simulink model "hpt_v2_topology2_paper"  (R2025a)
settings: Solver=ode23tb  StartTime=0.0  StopTime=0.2  RelTol=1e-3
model workspace (MAT data in the model file):
  hpt_ctrl_Ts = 2e-05
  hpt_energy_bridge_polarity = -1
  hpt_energy_control_sign = -1
  hpt_energy_i_ki = 100
  hpt_energy_i_kp = 0.5
  hpt_energy_id_max = 20
  hpt_energy_vff_gain = 1.06
  hpt_grid_f0 = 50
  hpt_inj_phase_offset = -1.05
  hpt_m_energy = 0
  hpt_m_energy_max = 0.95
  hpt_m_reg = 0.1
  hpt_m_reg_max = 0.8
  hpt_pll_ki = 2500
  hpt_pll_kp = 80
  hpt_pwm_fs = 2000
  hpt_reg_openloop_amp = 0
  hpt_reg_openloop_phase = 0
  hpt_reg_polarity = 1
  hpt_s2_resistance = 0.001
  hpt_sac_actor_select_mode = 0
  hpt_sac_dynamic_reg_limit = 0.6
  hpt_sac_enable = 0
  hpt_sac_energy_enable = 0
  hpt_sac_energy_max = 0.95
  hpt_sac_fixed_energy_d = 0
  hpt_sac_fixed_energy_q = 0
  hpt_sac_fixed_reg_d = 0
  hpt_sac_fixed_reg_q = 0
  hpt_sac_guard_enable = 0
  hpt_sac_i_base_peak = 816.496580928
  hpt_sac_policy_mode = 0
  hpt_sac_reg_d_gain = 1
  hpt_sac_reg_max = 0.8
  hpt_sac_reg_polarity = 1
  hpt_sac_reg_q_gain = 1
  hpt_sac_topology_id = 2
  hpt_sac_vdc_ref = 800
  hpt_sac_vref_phase = 230
  hpt_swell_gain_scale = 1
  hpt_swell_m_reg_max = 0.5
  hpt_swell_phase_offset = -0.5
  hpt_vdc_ki = 0.2
  hpt_vdc_kp = 2
  hpt_vdc_ref = 800
  hpt_vref_lv = 207
  hpt_vreg_ki = 0
  hpt_vreg_kp = 20
libraries: spsSeriesRLCBranchLib x17, simulink x9, spsLinearTransformerLib x9, spsVoltageMeasurementLib x7, spsGroundLib x5, spsUniversalBridgeLib x4, spsThreePhaseVIMeasurementLib x3, spsIGBTLib x1, spsThreePhaseSourceLib x1, spsThreePhaseSeriesRLCLoadLib x1, spsThreePhaseSeriesRLCBranchLib x1, spspowerguiLib x1
(part 1 of 2)
settings Model: Creator=m1391  LastModifiedBy=m1391

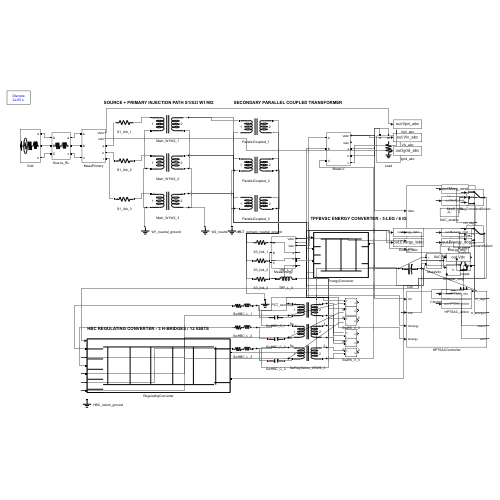
[thumbnail: Simulink's stored preview of the top-level diagram]
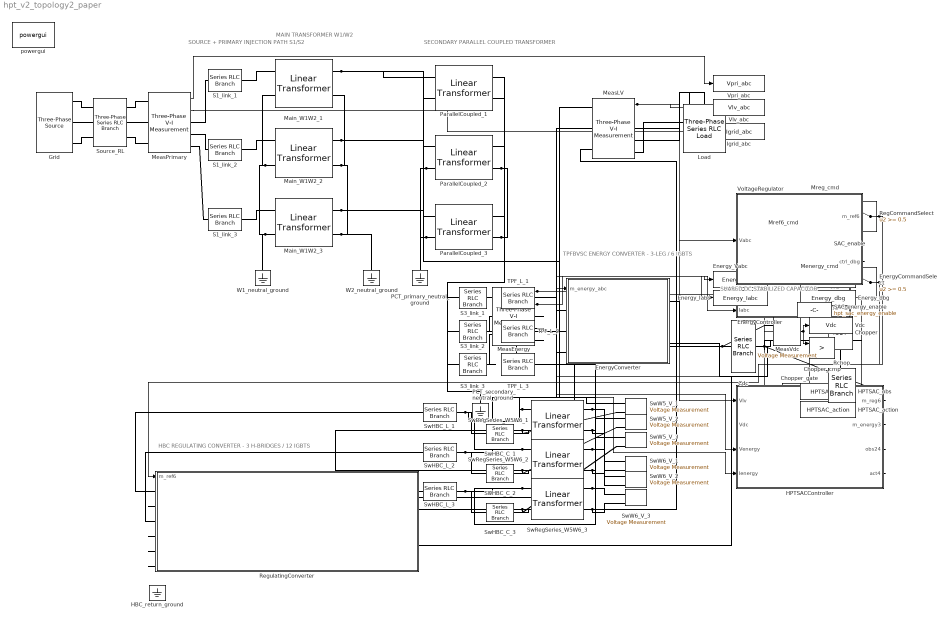
== system hpt_v2_topology2_paper ==
  note: SOURCE + PRIMARY INJECTION PATH S1/S2
  note: MAIN TRANSFORMER W1/W2
  note: SECONDARY PARALLEL COUPLED TRANSFORMER
  note: HBC REGULATING CONVERTER - 3 H-BRIDGES / 12 IGBTS
  note: TPFBVSC ENERGY CONVERTER - 3-LEG / 6 IGBTS
  note: SHARED DC STABILIZED CAPACITOR
  Cdc : spsSeriesRLCBranchLib/Series RLC Branch  LConnTagsString=__new0  RConnTagsString=__new0  BranchType=C  Resistance=1  Inductance=1e-3  SetiL0=off  InitialCurrent=0  Capacitance=0.0022  Setx0=on  InitialVoltage=800  Measurements=None
  Chopper : spsIGBTLib/IGBT  Ron=0.001  Lon=0  Vf=1  Tf=1e-6  Tt=2e-6  IC=0  Rs=1e5  Cs=inf  Measurements=on
  Chopper_cmp : RelationalOperator  Operator=>  OutDataTypeStr=boolean  RndMeth=Simplest  InputSameDT=off
  Chopper_gate : Constant  Value=850
  EnergyCommandSelect : Switch  Threshold=0.5  SaturateOnIntegerOverflow=off  InputSameDT=off
  EnergyController : Subsystem
  EnergyConverter : Subsystem
      mask Display:
      | color('black');
      | plot([10 90 90 10 10],[10 10 90 90 10]);
      | plot([20 80],[78 78]); plot([20 80],[22 22]);
      | plot([28 28],[22 78]); plot([50 50],[22 78]); plot([72 72],[22 78]);
      | plot([10 20],[65 65]); plot([10 20],[50 50]); plot([10 20],[35 35]);
      | plot([80 90],[65 65]); plot([80 90],[35 35]);
  Energy_Iabc : ToWorkspace  VariableName=Energy_Iabc  SampleTime=2e-05
  Energy_Vabc : ToWorkspace  VariableName=Energy_Vabc  SampleTime=2e-05
  Energy_dbg : ToWorkspace  VariableName=Energy_dbg  SampleTime=2e-05
  Grid : spsThreePhaseSourceLib/Three-Phase Source  InternalConnection=Yg  VoltagePhases=off  Voltage=10000  PhaseAngle=0  Voltage_phases=[25e3 25e3 25e3]/sqrt(3)  PhaseAngles_phases=[0 -120 +120]  Frequency=50  NonIdealSource=on  SpecifyImpedance=off  Resistance=0.8929  Inductance=16.58e-3  ShortCircuitLevel=100e6  BaseVoltage=25e3  XRratio=7  BusType=swing  Pref=10e3  Qref=0  Prefabc=[10e3, 10e3, 10e3]  Qrefabc=[0, 0, 0]  Qmin=-inf  Qmax=inf
  HBC_return_ground : spsGroundLib/Ground  LConnTagsString=a
  HPTSACController : Subsystem
  HPTSAC_action : ToWorkspace  VariableName=HPTSAC_action  SampleTime=2e-05
  HPTSAC_obs : ToWorkspace  VariableName=HPTSAC_obs  SampleTime=2e-05
  Igrid_abc : ToWorkspace  VariableName=Igrid_abc  SampleTime=2e-05
  Load : spsThreePhaseSeriesRLCLoadLib/Three-Phase Series RLC Load  LConnTagsString=A|B|C  Configuration=Y (grounded)  NominalVoltage=400  Vabc=[1e3 1e3 1e3]  Vabcp=[1e3 1e3 1e3]  NominalFrequency=50  UnbalancedPower=off  ActivePower=400000  InductivePower=0  CapacitivePower=0  Pabc=[10e3 9e3 11e3]  QLabc=[100 90 110]  QCabc=[100 90 110]  Pabcp=[10e3 9e3 11e3]  QLabcp=[100 90 110]  QCabcp=[100 90 110]  Measurements=None  LoadType=constant Z
  Main_W1W2_1 : spsLinearTransformerLib/Linear Transformer  UNITS=pu  NominalPower=[133333.3333,50]  winding1=[5773.5027,0.005,0.025]  winding2=[230.9401,0.005,0.025]  ThreeWindings=off  winding3=[ 315e3 0.002 0.08 ]  RmLm=[ 500 500 ]  Measurements=None  DataType=off
  Main_W1W2_2 : spsLinearTransformerLib/Linear Transformer  UNITS=pu  NominalPower=[133333.3333,50]  winding1=[5773.5027,0.005,0.025]  winding2=[230.9401,0.005,0.025]  ThreeWindings=off  winding3=[ 315e3 0.002 0.08 ]  RmLm=[ 500 500 ]  Measurements=None  DataType=off
  Main_W1W2_3 : spsLinearTransformerLib/Linear Transformer  UNITS=pu  NominalPower=[133333.3333,50]  winding1=[5773.5027,0.005,0.025]  winding2=[230.9401,0.005,0.025]  ThreeWindings=off  winding3=[ 315e3 0.002 0.08 ]  RmLm=[ 500 500 ]  Measurements=None  DataType=off
  MeasEnergy : spsThreePhaseVIMeasurementLib/Three-Phase V-I Measurement  VoltageMeasurement=phase-to-ground  SetLabelV=off  LabelV=Vabc  Vpu=off  VpuLL=off  CurrentMeasurement=yes  SetLabelI=off  LabelI=Iabc  Ipu=off  Pbase=100e6  Vbase=500e3  OutputType=Complex  PhasorSimulation=off  PSBequivalent=0
  MeasLV : spsThreePhaseVIMeasurementLib/Three-Phase V-I Measurement  VoltageMeasurement=phase-to-ground  SetLabelV=off  LabelV=Vabc  Vpu=off  VpuLL=off  CurrentMeasurement=yes  SetLabelI=off  LabelI=Iabc  Ipu=off  Pbase=100e6  Vbase=500e3  OutputType=Complex  PhasorSimulation=off  PSBequivalent=0
  MeasPrimary : spsThreePhaseVIMeasurementLib/Three-Phase V-I Measurement  VoltageMeasurement=phase-to-ground  SetLabelV=off  LabelV=Vabc  Vpu=off  VpuLL=off  CurrentMeasurement=yes  SetLabelI=off  LabelI=Iabc  Ipu=off  Pbase=100e6  Vbase=500e3  OutputType=Complex  PhasorSimulation=off  PSBequivalent=0
  MeasVdc : spsVoltageMeasurementLib/Voltage Measurement  PhasorSimulation=off  OutputType=Complex  PSBequivalent=0
  Menergy_cmd : ToWorkspace  VariableName=Menergy_cmd  SampleTime=2e-05
  Mref6_cmd : ToWorkspace  VariableName=Mref6_cmd  SampleTime=2e-05
  Mreg_cmd : ToWorkspace  VariableName=Mreg_cmd  SampleTime=2e-05
  PCT_primary_neutral_ground : spsGroundLib/Ground  LConnTagsString=a
  PCT_secondary_neutral_ground : spsGroundLib/Ground  LConnTagsString=a
  ParallelCoupled_1 : spsLinearTransformerLib/Linear Transformer  UNITS=pu  NominalPower=[40000,50]  winding1=[230.9401,0.004,0.02]  winding2=[230.9401,0.004,0.02]  ThreeWindings=off  winding3=[ 315e3 0.002 0.08 ]  RmLm=[ 500 500 ]  Measurements=None  DataType=off
  ParallelCoupled_2 : spsLinearTransformerLib/Linear Transformer  UNITS=pu  NominalPower=[40000,50]  winding1=[230.9401,0.004,0.02]  winding2=[230.9401,0.004,0.02]  ThreeWindings=off  winding3=[ 315e3 0.002 0.08 ]  RmLm=[ 500 500 ]  Measurements=None  DataType=off
  ParallelCoupled_3 : spsLinearTransformerLib/Linear Transformer  UNITS=pu  NominalPower=[40000,50]  winding1=[230.9401,0.004,0.02]  winding2=[230.9401,0.004,0.02]  ThreeWindings=off  winding3=[ 315e3 0.002 0.08 ]  RmLm=[ 500 500 ]  Measurements=None  DataType=off
  Rchop : spsSeriesRLCBranchLib/Series RLC Branch  LConnTagsString=__new0  RConnTagsString=__new0  BranchType=R  Resistance=5.3333  Inductance=1e-3  SetiL0=off  InitialCurrent=0  Capacitance=1e-6  Setx0=off  InitialVoltage=0  Measurements=None
  RegCommandSelect : Switch  Threshold=0.5  SaturateOnIntegerOverflow=off  InputSameDT=off
  RegulatingConverter : Subsystem
      mask Display:
      | color('black');
      | plot([5 95 95 5 5],[10 10 90 90 10]);
      | plot([15 85],[78 78]); plot([15 85],[22 22]);
      | plot([18 18],[22 78]); plot([32 32],[22 78]);
      | plot([45 45],[22 78]); plot([59 59],[22 78]);
      | plot([72 72],[22 78]); plot([86 86],[22 78]);
      | plot([5 15],[75 75]); plot([5 15],[60 60]); plot([5 15],[45 45]);
      | plot([5 15],[30 30]); plot([5 15],[15 15]); plot([5 15],[10 10]);
      | plot([85 95],[75 75]); plot([85 95],[25 25]);
  S1_link_1 : spsSeriesRLCBranchLib/Series RLC Branch  LConnTagsString=__new0  RConnTagsString=__new0  BranchType=R  Resistance=1e-3  Inductance=1e-3  SetiL0=off  InitialCurrent=0  Capacitance=1e-6  Setx0=off  InitialVoltage=0  Measurements=None
  S1_link_2 : spsSeriesRLCBranchLib/Series RLC Branch  LConnTagsString=__new0  RConnTagsString=__new0  BranchType=R  Resistance=1e-3  Inductance=1e-3  SetiL0=off  InitialCurrent=0  Capacitance=1e-6  Setx0=off  InitialVoltage=0  Measurements=None
  S1_link_3 : spsSeriesRLCBranchLib/Series RLC Branch  LConnTagsString=__new0  RConnTagsString=__new0  BranchType=R  Resistance=1e-3  Inductance=1e-3  SetiL0=off  InitialCurrent=0  Capacitance=1e-6  Setx0=off  InitialVoltage=0  Measurements=None
  S3_link_1 : spsSeriesRLCBranchLib/Series RLC Branch  LConnTagsString=__new0  RConnTagsString=__new0  BranchType=R  Resistance=1e-3  Inductance=1e-3  SetiL0=off  InitialCurrent=0  Capacitance=1e-6  Setx0=off  InitialVoltage=0  Measurements=None
  S3_link_2 : spsSeriesRLCBranchLib/Series RLC Branch  LConnTagsString=__new0  RConnTagsString=__new0  BranchType=R  Resistance=1e-3  Inductance=1e-3  SetiL0=off  InitialCurrent=0  Capacitance=1e-6  Setx0=off  InitialVoltage=0  Measurements=None
  S3_link_3 : spsSeriesRLCBranchLib/Series RLC Branch  LConnTagsString=__new0  RConnTagsString=__new0  BranchType=R  Resistance=1e-3  Inductance=1e-3  SetiL0=off  InitialCurrent=0  Capacitance=1e-6  Setx0=off  InitialVoltage=0  Measurements=None
  SAC_enable : Constant  Value=hpt_sac_enable
  SAC_energy_enable : Constant  Value=hpt_sac_energy_enable
  Source_RL : spsThreePhaseSeriesRLCBranchLib/Three-Phase Series RLC Branch  LConnTagsString=A|B|C  RConnTagsString=A|B|C  BranchType=RL  Resistance=11.7851  Inductance=0.26259  Capacitance=1e-6  Measurements=None
  SwHBC_C_1 : spsSeriesRLCBranchLib/Series RLC Branch  LConnTagsString=__new0  RConnTagsString=__new0  BranchType=C  Resistance=1  Inductance=1e-3  SetiL0=off  InitialCurrent=0  Capacitance=2e-05  Setx0=off  InitialVoltage=0  Measurements=None
  SwHBC_C_2 : spsSeriesRLCBranchLib/Series RLC Branch  LConnTagsString=__new0  RConnTagsString=__new0  BranchType=C  Resistance=1  Inductance=1e-3  SetiL0=off  InitialCurrent=0  Capacitance=2e-05  Setx0=off  InitialVoltage=0  Measurements=None
  SwHBC_C_3 : spsSeriesRLCBranchLib/Series RLC Branch  LConnTagsString=__new0  RConnTagsString=__new0  BranchType=C  Resistance=1  Inductance=1e-3  SetiL0=off  InitialCurrent=0  Capacitance=2e-05  Setx0=off  InitialVoltage=0  Measurements=None
  SwHBC_L_1 : spsSeriesRLCBranchLib/Series RLC Branch  LConnTagsString=__new0  RConnTagsString=__new0  BranchType=RL  Resistance=0.03  Inductance=0.002  SetiL0=off  InitialCurrent=0  Capacitance=1e-6  Setx0=off  InitialVoltage=0  Measurements=None
  SwHBC_L_2 : spsSeriesRLCBranchLib/Series RLC Branch  LConnTagsString=__new0  RConnTagsString=__new0  BranchType=RL  Resistance=0.03  Inductance=0.002  SetiL0=off  InitialCurrent=0  Capacitance=1e-6  Setx0=off  InitialVoltage=0  Measurements=None
  SwHBC_L_3 : spsSeriesRLCBranchLib/Series RLC Branch  LConnTagsString=__new0  RConnTagsString=__new0  BranchType=RL  Resistance=0.03  Inductance=0.002  SetiL0=off  InitialCurrent=0  Capacitance=1e-6  Setx0=off  InitialVoltage=0  Measurements=None
  SwRegSeries_W5W6_1 : spsLinearTransformerLib/Linear Transformer  UNITS=pu  NominalPower=[30000,50]  winding1=[400,0.002,0.03]  winding2=[100,0.002,0.03]  ThreeWindings=off  winding3=[ 315e3 0.002 0.08 ]  RmLm=[ 500 500 ]  Measurements=None  DataType=off
  SwRegSeries_W5W6_2 : spsLinearTransformerLib/Linear Transformer  UNITS=pu  NominalPower=[30000,50]  winding1=[400,0.002,0.03]  winding2=[100,0.002,0.03]  ThreeWindings=off  winding3=[ 315e3 0.002 0.08 ]  RmLm=[ 500 500 ]  Measurements=None  DataType=off
  SwRegSeries_W5W6_3 : spsLinearTransformerLib/Linear Transformer  UNITS=pu  NominalPower=[30000,50]  winding1=[400,0.002,0.03]  winding2=[100,0.002,0.03]  ThreeWindings=off  winding3=[ 315e3 0.002 0.08 ]  RmLm=[ 500 500 ]  Measurements=None  DataType=off
  SwW5_V_1 : spsVoltageMeasurementLib/Voltage Measurement  PhasorSimulation=off  OutputType=Complex  PSBequivalent=0
  SwW5_V_2 : spsVoltageMeasurementLib/Voltage Measurement  PhasorSimulation=off  OutputType=Complex  PSBequivalent=0
  SwW5_V_3 : spsVoltageMeasurementLib/Voltage Measurement  PhasorSimulation=off  OutputType=Complex  PSBequivalent=0
  SwW6_V_1 : spsVoltageMeasurementLib/Voltage Measurement  PhasorSimulation=off  OutputType=Complex  PSBequivalent=0
  SwW6_V_2 : spsVoltageMeasurementLib/Voltage Measurement  PhasorSimulation=off  OutputType=Complex  PSBequivalent=0
  SwW6_V_3 : spsVoltageMeasurementLib/Voltage Measurement  PhasorSimulation=off  OutputType=Complex  PSBequivalent=0
  TPF_L_1 : spsSeriesRLCBranchLib/Series RLC Branch  LConnTagsString=__new0  RConnTagsString=__new0  BranchType=L  Resistance=1  Inductance=0.0015  SetiL0=off  InitialCurrent=0  Capacitance=1e-6  Setx0=off  InitialVoltage=0  Measurements=None
  TPF_L_2 : spsSeriesRLCBranchLib/Series RLC Branch  LConnTagsString=__new0  RConnTagsString=__new0  BranchType=L  Resistance=1  Inductance=0.0015  SetiL0=off  InitialCurrent=0  Capacitance=1e-6  Setx0=off  InitialVoltage=0  Measurements=None
  TPF_L_3 : spsSeriesRLCBranchLib/Series RLC Branch  LConnTagsString=__new0  RConnTagsString=__new0  BranchType=L  Resistance=1  Inductance=0.0015  SetiL0=off  InitialCurrent=0  Capacitance=1e-6  Setx0=off  InitialVoltage=0  Measurements=None
  Vdc : ToWorkspace  VariableName=Vdc  SampleTime=2e-05
  Vlv_abc : ToWorkspace  VariableName=Vlv_abc  SampleTime=2e-05
  VoltageRegulator : Subsystem
  Vpri_abc : ToWorkspace  VariableName=Vpri_abc  SampleTime=2e-05
  W1_neutral_ground : spsGroundLib/Ground  LConnTagsString=a
  W2_neutral_ground : spsGroundLib/Ground  LConnTagsString=a
  powergui : spspowerguiLib/powergui  Priority=1  SimulationMode=Discrete  SampleTime=2e-05  frequency=60  Iterations=50  frequencyindice=60  Pbase=100e6  ErrMax=1e-4  UnitsV=kV  UnitsW=MW  buscounter=0  FunctionMessages=off  echomessages=off  EnableUseOfTLC=off  CurrentSourceSwitches=off  DisableSnubberDevices=off  DisableRonSwitches=off  DisableVfSwitches=off  DisplayEquations=off  AutomaticDiscreteSolvers=off  SolverType=Tustin/Backward Euler (TBE)  Interpol=off  ExternalGateDelay=off  methode=off  Ts=100  x0status=blocks  SPID=on  SwTol=0  HookPort=off  NonlinearTolerance=1e-4  nMaxIteration=100  ContinueOnMaxIteration=off  RestoreLinks=warning  ResistiveCurrentMeasurement=off  Frange=[0:2:500]  Ylog=off  Xlog=on  ShowGrid=off  save=off  variable=ZData  structure=0  ZoomFFT=off  StartTime=0.0  cycles=1  DisplayStyle=1  fundamental=60  FreqAxis=off  MaxFrequency=1000  frequencyindicesteady=1  RmsSteady=1  display=off
  wires:
  MeasVdc/1 -> Chopper_cmp/1, Vdc/1, HPTSACController/2(Vdc), EnergyController/1(Vdc)
  Chopper_gate/1 -> Chopper_cmp/2
  Chopper_cmp/1 -> Chopper/1
  MeasPrimary/1 -> Vpri_abc/1
  MeasPrimary/2 -> Igrid_abc/1
  MeasLV/1 -> Vlv_abc/1, VoltageRegulator/1(Vabc), HPTSACController/1(Vlv)
  VoltageRegulator/1(m_ref6) -> RegCommandSelect/3
  HPTSACController/1(m_reg6) -> RegCommandSelect/1
  SAC_enable/1 -> RegCommandSelect/2
  RegCommandSelect/1 -> RegulatingConverter/1(m_ref6), Mref6_cmd/1
  VoltageRegulator/2(ctrl_dbg) -> Mreg_cmd/1
  MeasEnergy/1 -> EnergyController/2(Vabc), HPTSACController/3(Venergy), Energy_Vabc/1
  MeasEnergy/2 -> EnergyController/3(Iabc), HPTSACController/4(Ienergy), Energy_Iabc/1
  EnergyController/1(m_energy_abc) -> EnergyCommandSelect/3
  HPTSACController/2(m_energy3) -> EnergyCommandSelect/1
  SAC_energy_enable/1 -> EnergyCommandSelect/2
  EnergyCommandSelect/1 -> EnergyConverter/1(m_energy_abc), Menergy_cmd/1
  EnergyController/2(energy_dbg) -> Energy_dbg/1
  HPTSACController/3(obs24) -> HPTSAC_obs/1
  HPTSACController/4(act4) -> HPTSAC_action/1
  connections:
  Grid/RConn1 -- Source_RL/LConn1
  Source_RL/RConn1 -- MeasPrimary/LConn1
  MeasPrimary/RConn1 -- S1_link_1/LConn1
  S1_link_1/RConn1 -- Main_W1W2_1/LConn1
  ParallelCoupled_1/LConn1 -- Main_W1W2_1/RConn1 -- SwRegSeries_W5W6_1/RConn1 -- SwW6_V_1/LConn1
  MeasLV/LConn1 -- SwRegSeries_W5W6_1/RConn2 -- SwW6_V_1/LConn2
  MeasLV/RConn1 -- Load/LConn1
  ParallelCoupled_1/RConn1 -- S3_link_1/LConn1
  S3_link_1/RConn1 -- MeasEnergy/LConn1
  MeasEnergy/RConn1 -- TPF_L_1/LConn1
  TPF_L_1/RConn1 -- EnergyConverter/LConn1
  RegulatingConverter/LConn1 -- SwHBC_L_1/LConn1
  SwHBC_L_1/RConn1 -- SwHBC_C_1/LConn1 -- SwRegSeries_W5W6_1/LConn1 -- SwW5_V_1/LConn1
  RegulatingConverter/LConn2 -- SwHBC_C_1/RConn1 -- SwRegSeries_W5W6_1/LConn2 -- SwW5_V_1/LConn2
  Grid/RConn2 -- Source_RL/LConn2
  Source_RL/RConn2 -- MeasPrimary/LConn2
  MeasPrimary/RConn2 -- S1_link_2/LConn1
  S1_link_2/RConn1 -- Main_W1W2_2/LConn1
  ParallelCoupled_2/LConn1 -- Main_W1W2_2/RConn1 -- SwRegSeries_W5W6_2/RConn1 -- SwW6_V_2/LConn1
  MeasLV/LConn2 -- SwRegSeries_W5W6_2/RConn2 -- SwW6_V_2/LConn2
  MeasLV/RConn2 -- Load/LConn2
  ParallelCoupled_2/RConn1 -- S3_link_2/LConn1
  S3_link_2/RConn1 -- MeasEnergy/LConn2
  MeasEnergy/RConn2 -- TPF_L_2/LConn1
  TPF_L_2/RConn1 -- EnergyConverter/LConn2
  RegulatingConverter/LConn3 -- SwHBC_L_2/LConn1
  SwHBC_L_2/RConn1 -- SwHBC_C_2/LConn1 -- SwRegSeries_W5W6_2/LConn1 -- SwW5_V_2/LConn1
  RegulatingConverter/LConn4 -- SwHBC_C_2/RConn1 -- SwRegSeries_W5W6_2/LConn2 -- SwW5_V_2/LConn2
  Grid/RConn3 -- Source_RL/LConn3
  Source_RL/RConn3 -- MeasPrimary/LConn3
  MeasPrimary/RConn3 -- S1_link_3/LConn1
  S1_link_3/RConn1 -- Main_W1W2_3/LConn1
  ParallelCoupled_3/LConn1 -- Main_W1W2_3/RConn1 -- SwRegSeries_W5W6_3/RConn1 -- SwW6_V_3/LConn1
  MeasLV/LConn3 -- SwRegSeries_W5W6_3/RConn2 -- SwW6_V_3/LConn2
  MeasLV/RConn3 -- Load/LConn3
  ParallelCoupled_3/RConn1 -- S3_link_3/LConn1
  S3_link_3/RConn1 -- MeasEnergy/LConn3
  MeasEnergy/RConn3 -- TPF_L_3/LConn1
  TPF_L_3/RConn1 -- EnergyConverter/LConn3
  RegulatingConverter/LConn5 -- SwHBC_L_3/LConn1
  SwHBC_L_3/RConn1 -- SwHBC_C_3/LConn1 -- SwRegSeries_W5W6_3/LConn1 -- SwW5_V_3/LConn1
  RegulatingConverter/LConn6 -- SwHBC_C_3/RConn1 -- SwRegSeries_W5W6_3/LConn2 -- SwW5_V_3/LConn2
  Main_W1W2_2/LConn2 -- Main_W1W2_1/LConn2 -- Main_W1W2_3/LConn2 -- W1_neutral_ground/LConn1
  Main_W1W2_2/RConn2 -- Main_W1W2_1/RConn2 -- Main_W1W2_3/RConn2 -- W2_neutral_ground/LConn1
  ParallelCoupled_2/LConn2 -- ParallelCoupled_1/LConn2 -- ParallelCoupled_3/LConn2 -- PCT_primary_neutral_ground/LConn1
  ParallelCoupled_2/RConn2 -- ParallelCoupled_1/RConn2 -- ParallelCoupled_3/RConn2 -- PCT_secondary_neutral_ground/LConn1
  EnergyConverter/RConn1 -- Cdc/LConn1 -- RegulatingConverter/RConn1 -- MeasVdc/LConn1 -- Chopper/LConn1
  EnergyConverter/RConn2 -- RegulatingConverter/RConn2 -- MeasVdc/LConn2 -- Cdc/RConn1 -- Rchop/RConn1
  Chopper/RConn1 -- Rchop/LConn1

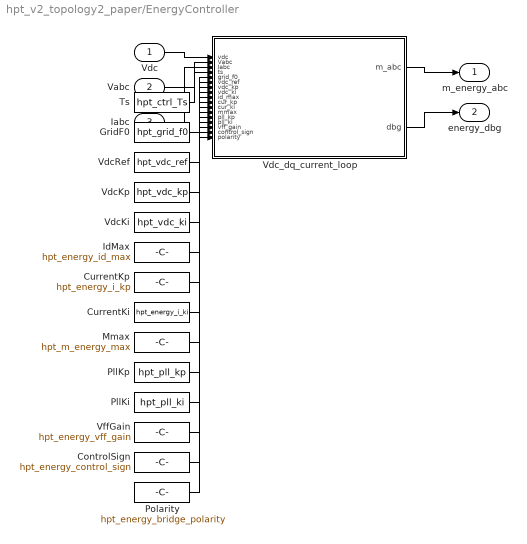
== system hpt_v2_topology2_paper/EnergyController ==
  Vdc : Inport
  Vabc : Inport  Port=2
  Iabc : Inport  Port=3
  ControlSign : Constant  Value=hpt_energy_control_sign
  CurrentKi : Constant  Value=hpt_energy_i_ki
  CurrentKp : Constant  Value=hpt_energy_i_kp
  GridF0 : Constant  Value=hpt_grid_f0
  IdMax : Constant  Value=hpt_energy_id_max
  Mmax : Constant  Value=hpt_m_energy_max
  PllKi : Constant  Value=hpt_pll_ki
  PllKp : Constant  Value=hpt_pll_kp
  Polarity : Constant  Value=hpt_energy_bridge_polarity
  Ts : Constant  Value=hpt_ctrl_Ts
  VdcKi : Constant  Value=hpt_vdc_ki
  VdcKp : Constant  Value=hpt_vdc_kp
  VdcRef : Constant  Value=hpt_vdc_ref
  Vdc_dq_current_loop : MATLAB Function  TreatAsAtomicUnit=on
  VffGain : Constant  Value=hpt_energy_vff_gain
  m_energy_abc : Outport
  energy_dbg : Outport  Port=2
  wires:
  Ts/1 -> Vdc_dq_current_loop/4(ts)
  GridF0/1 -> Vdc_dq_current_loop/5(grid_f0)
  VdcRef/1 -> Vdc_dq_current_loop/6(vdc_ref)
  VdcKp/1 -> Vdc_dq_current_loop/7(vdc_kp)
  VdcKi/1 -> Vdc_dq_current_loop/8(vdc_ki)
  IdMax/1 -> Vdc_dq_current_loop/9(id_max)
  CurrentKp/1 -> Vdc_dq_current_loop/10(cur_kp)
  CurrentKi/1 -> Vdc_dq_current_loop/11(cur_ki)
  Mmax/1 -> Vdc_dq_current_loop/12(mmax)
  PllKp/1 -> Vdc_dq_current_loop/13(pll_kp)
  PllKi/1 -> Vdc_dq_current_loop/14(pll_ki)
  VffGain/1 -> Vdc_dq_current_loop/15(vff_gain)
  ControlSign/1 -> Vdc_dq_current_loop/16(control_sign)
  Polarity/1 -> Vdc_dq_current_loop/17(polarity)
  Vdc/1 -> Vdc_dq_current_loop/1(vdc)
  Vabc/1 -> Vdc_dq_current_loop/2(Vabc)
  Iabc/1 -> Vdc_dq_current_loop/3(Iabc)
  Vdc_dq_current_loop/1(m_abc) -> m_energy_abc/1
  Vdc_dq_current_loop/2(dbg) -> energy_dbg/1

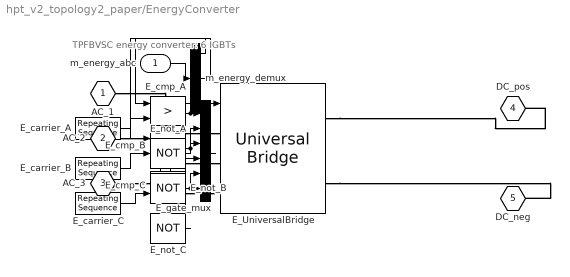
== system hpt_v2_topology2_paper/EnergyConverter ==
  note: TPFBVSC energy converter: 6 IGBTs
  m_energy_abc : Inport
  E_UniversalBridge : spsUniversalBridgeLib/Universal Bridge  Arms=3  SnubberResistance=1e5  SnubberCapacitance=inf  Device=IGBT / Diodes  Ron=1e-3  Lon=0  ForwardVoltages=[0.8 0.8]  ForwardVoltage=0  GTOparameters=[ 10e-6 , 20e-6 ]  IGBTparameters=[ 1e-6 , 2e-6 ]  Measurements=None  Measurements_2=None  converterType=Rectifier
  E_carrier_A : simulink/Sources/Repeating Sequence  rep_seq_t=[0 0.5/hpt_pwm_fs 1/hpt_pwm_fs]  rep_seq_y=[-1 1 -1]
  E_carrier_B : simulink/Sources/Repeating Sequence  rep_seq_t=[0 0.5/hpt_pwm_fs 1/hpt_pwm_fs]  rep_seq_y=[-1 1 -1]
  E_carrier_C : simulink/Sources/Repeating Sequence  rep_seq_t=[0 0.5/hpt_pwm_fs 1/hpt_pwm_fs]  rep_seq_y=[-1 1 -1]
  E_cmp_A : RelationalOperator  Operator=>  OutDataTypeStr=boolean  RndMeth=Simplest  InputSameDT=off
  E_cmp_B : RelationalOperator  Operator=>  OutDataTypeStr=boolean  RndMeth=Simplest  InputSameDT=off
  E_cmp_C : RelationalOperator  Operator=>  OutDataTypeStr=boolean  RndMeth=Simplest  InputSameDT=off
  E_gate_mux : Mux  Inputs=6
  E_not_A : Logic  Operator=NOT  AllPortsSameDT=off  OutDataTypeStr=boolean
  E_not_B : Logic  Operator=NOT  AllPortsSameDT=off  OutDataTypeStr=boolean
  E_not_C : Logic  Operator=NOT  AllPortsSameDT=off  OutDataTypeStr=boolean
  m_energy_demux : Demux  Outputs=3
  AC_1 : PMIOPort  Side=Left
  AC_2 : PMIOPort  Port=2  Side=Left
  AC_3 : PMIOPort  Port=3  Side=Left
  DC_pos : PMIOPort  Port=4  Side=Right
  DC_neg : PMIOPort  Port=5  Side=Right
  wires:
  m_energy_abc/1 -> m_energy_demux/1
  m_energy_demux/1 -> E_cmp_A/1
  E_carrier_A/1 -> E_cmp_A/2
  E_cmp_A/1 -> E_gate_mux/1, E_not_A/1
  E_not_A/1 -> E_gate_mux/2
  m_energy_demux/2 -> E_cmp_B/1
  E_carrier_B/1 -> E_cmp_B/2
  E_cmp_B/1 -> E_gate_mux/3, E_not_B/1
  E_not_B/1 -> E_gate_mux/4
  m_energy_demux/3 -> E_cmp_C/1
  E_carrier_C/1 -> E_cmp_C/2
  E_cmp_C/1 -> E_gate_mux/5, E_not_C/1
  E_not_C/1 -> E_gate_mux/6
  E_gate_mux/1 -> E_UniversalBridge/1
  connections:
  AC_1/RConn1 -- E_UniversalBridge/LConn1
  AC_2/RConn1 -- E_UniversalBridge/LConn2
  AC_3/RConn1 -- E_UniversalBridge/LConn3
  E_UniversalBridge/RConn1 -- DC_pos/RConn1
  E_UniversalBridge/RConn2 -- DC_neg/RConn1

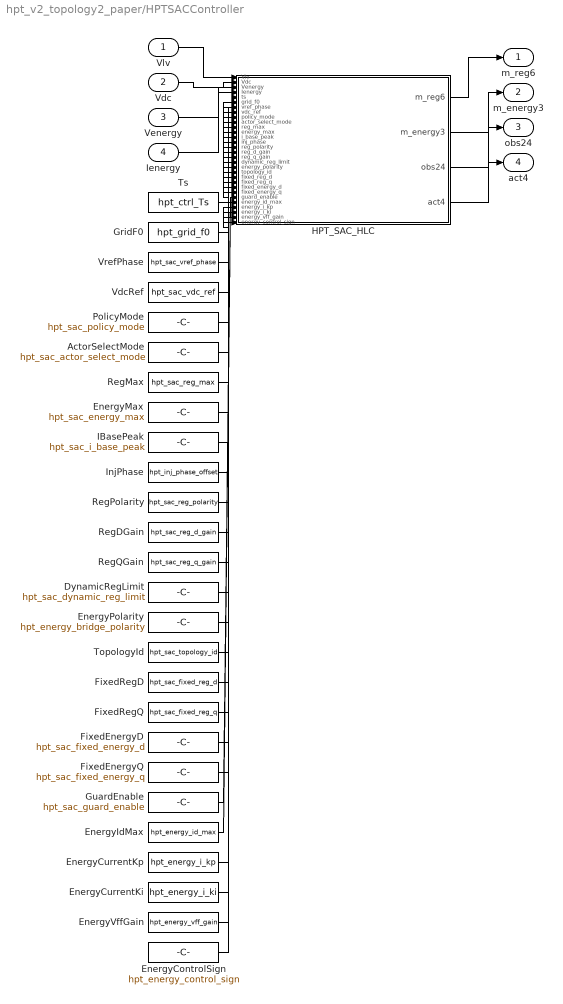
== system hpt_v2_topology2_paper/HPTSACController ==
  Vlv : Inport
  Vdc : Inport  Port=2
  Venergy : Inport  Port=3
  Ienergy : Inport  Port=4
  ActorSelectMode : Constant  Value=hpt_sac_actor_select_mode
  DynamicRegLimit : Constant  Value=hpt_sac_dynamic_reg_limit
  EnergyControlSign : Constant  Value=hpt_energy_control_sign
  EnergyCurrentKi : Constant  Value=hpt_energy_i_ki
  EnergyCurrentKp : Constant  Value=hpt_energy_i_kp
  EnergyIdMax : Constant  Value=hpt_energy_id_max
  EnergyMax : Constant  Value=hpt_sac_energy_max
  EnergyPolarity : Constant  Value=hpt_energy_bridge_polarity
  EnergyVffGain : Constant  Value=hpt_energy_vff_gain
  FixedEnergyD : Constant  Value=hpt_sac_fixed_energy_d
  FixedEnergyQ : Constant  Value=hpt_sac_fixed_energy_q
  FixedRegD : Constant  Value=hpt_sac_fixed_reg_d
  FixedRegQ : Constant  Value=hpt_sac_fixed_reg_q
  GridF0 : Constant  Value=hpt_grid_f0
  GuardEnable : Constant  Value=hpt_sac_guard_enable
  HPT_SAC_HLC : MATLAB Function  TreatAsAtomicUnit=on
  IBasePeak : Constant  Value=hpt_sac_i_base_peak
  InjPhase : Constant  Value=hpt_inj_phase_offset
  PolicyMode : Constant  Value=hpt_sac_policy_mode
  RegDGain : Constant  Value=hpt_sac_reg_d_gain
  RegMax : Constant  Value=hpt_sac_reg_max
  RegPolarity : Constant  Value=hpt_sac_reg_polarity
  RegQGain : Constant  Value=hpt_sac_reg_q_gain
  TopologyId : Constant  Value=hpt_sac_topology_id
  Ts : Constant  Value=hpt_ctrl_Ts
  VdcRef : Constant  Value=hpt_sac_vdc_ref
  VrefPhase : Constant  Value=hpt_sac_vref_phase
  m_reg6 : Outport
  m_energy3 : Outport  Port=2
  obs24 : Outport  Port=3
  act4 : Outport  Port=4
  wires:
  Ts/1 -> HPT_SAC_HLC/5(ts)
  GridF0/1 -> HPT_SAC_HLC/6(grid_f0)
  VrefPhase/1 -> HPT_SAC_HLC/7(vref_phase)
  VdcRef/1 -> HPT_SAC_HLC/8(vdc_ref)
  PolicyMode/1 -> HPT_SAC_HLC/9(policy_mode)
  ActorSelectMode/1 -> HPT_SAC_HLC/10(actor_select_mode)
  RegMax/1 -> HPT_SAC_HLC/11(reg_max)
  EnergyMax/1 -> HPT_SAC_HLC/12(energy_max)
  IBasePeak/1 -> HPT_SAC_HLC/13(i_base_peak)
  InjPhase/1 -> HPT_SAC_HLC/14(inj_phase)
  RegPolarity/1 -> HPT_SAC_HLC/15(reg_polarity)
  RegDGain/1 -> HPT_SAC_HLC/16(reg_d_gain)
  RegQGain/1 -> HPT_SAC_HLC/17(reg_q_gain)
  DynamicRegLimit/1 -> HPT_SAC_HLC/18(dynamic_reg_limit)
  EnergyPolarity/1 -> HPT_SAC_HLC/19(energy_polarity)
  TopologyId/1 -> HPT_SAC_HLC/20(topology_id)
  FixedRegD/1 -> HPT_SAC_HLC/21(fixed_reg_d)
  FixedRegQ/1 -> HPT_SAC_HLC/22(fixed_reg_q)
  FixedEnergyD/1 -> HPT_SAC_HLC/23(fixed_energy_d)
  FixedEnergyQ/1 -> HPT_SAC_HLC/24(fixed_energy_q)
  GuardEnable/1 -> HPT_SAC_HLC/25(guard_enable)
  EnergyIdMax/1 -> HPT_SAC_HLC/26(energy_id_max)
  EnergyCurrentKp/1 -> HPT_SAC_HLC/27(energy_i_kp)
  EnergyCurrentKi/1 -> HPT_SAC_HLC/28(energy_i_ki)
  EnergyVffGain/1 -> HPT_SAC_HLC/29(energy_vff_gain)
  EnergyControlSign/1 -> HPT_SAC_HLC/30(energy_control_sign)
  Vlv/1 -> HPT_SAC_HLC/1(Vlv)
  Vdc/1 -> HPT_SAC_HLC/2(Vdc)
  Venergy/1 -> HPT_SAC_HLC/3(Venergy)
  Ienergy/1 -> HPT_SAC_HLC/4(Ienergy)
  HPT_SAC_HLC/1(m_reg6) -> m_reg6/1
  HPT_SAC_HLC/2(m_energy3) -> m_energy3/1
  HPT_SAC_HLC/3(obs24) -> obs24/1
  HPT_SAC_HLC/4(act4) -> act4/1

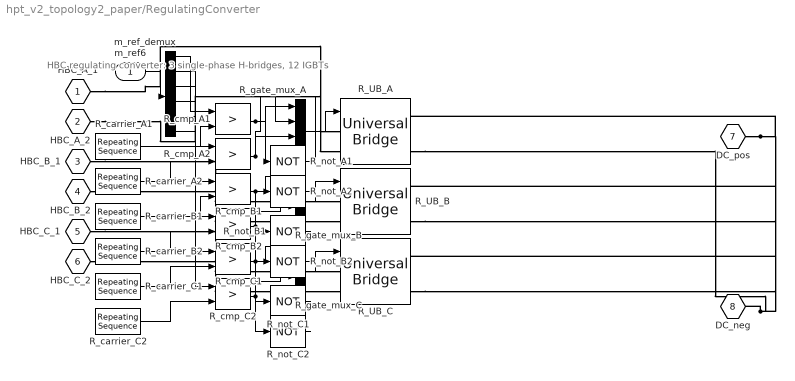
== system hpt_v2_topology2_paper/RegulatingConverter ==
  note: HBC regulating converter: 3 single-phase H-bridges, 12 IGBTs
  m_ref6 : Inport
  R_UB_A : spsUniversalBridgeLib/Universal Bridge  Arms=2  SnubberResistance=1e5  SnubberCapacitance=1e-9  Device=IGBT / Diodes  Ron=1e-3  Lon=0  ForwardVoltages="[  0  0  ]"  ForwardVoltage=0  GTOparameters=[ 10e-6 , 20e-6 ]  IGBTparameters=[ 1e-6 , 2e-6 ]  Measurements=None  Measurements_2=None  converterType=Rectifier
  R_UB_B : spsUniversalBridgeLib/Universal Bridge  Arms=2  SnubberResistance=1e5  SnubberCapacitance=1e-9  Device=IGBT / Diodes  Ron=1e-3  Lon=0  ForwardVoltages="[  0  0  ]"  ForwardVoltage=0  GTOparameters=[ 10e-6 , 20e-6 ]  IGBTparameters=[ 1e-6 , 2e-6 ]  Measurements=None  Measurements_2=None  converterType=Rectifier
  R_UB_C : spsUniversalBridgeLib/Universal Bridge  Arms=2  SnubberResistance=1e5  SnubberCapacitance=1e-9  Device=IGBT / Diodes  Ron=1e-3  Lon=0  ForwardVoltages="[  0  0  ]"  ForwardVoltage=0  GTOparameters=[ 10e-6 , 20e-6 ]  IGBTparameters=[ 1e-6 , 2e-6 ]  Measurements=None  Measurements_2=None  converterType=Rectifier
  R_carrier_A1 : simulink/Sources/Repeating Sequence  rep_seq_t=[0 0.5/hpt_pwm_fs 1/hpt_pwm_fs]  rep_seq_y=[-1 1 -1]
  R_carrier_A2 : simulink/Sources/Repeating Sequence  rep_seq_t=[0 0.5/hpt_pwm_fs 1/hpt_pwm_fs]  rep_seq_y=[-1 1 -1]
  R_carrier_B1 : simulink/Sources/Repeating Sequence  rep_seq_t=[0 0.5/hpt_pwm_fs 1/hpt_pwm_fs]  rep_seq_y=[-1 1 -1]
  R_carrier_B2 : simulink/Sources/Repeating Sequence  rep_seq_t=[0 0.5/hpt_pwm_fs 1/hpt_pwm_fs]  rep_seq_y=[-1 1 -1]
  R_carrier_C1 : simulink/Sources/Repeating Sequence  rep_seq_t=[0 0.5/hpt_pwm_fs 1/hpt_pwm_fs]  rep_seq_y=[-1 1 -1]
  R_carrier_C2 : simulink/Sources/Repeating Sequence  rep_seq_t=[0 0.5/hpt_pwm_fs 1/hpt_pwm_fs]  rep_seq_y=[-1 1 -1]
  R_cmp_A1 : RelationalOperator  Operator=>  OutDataTypeStr=boolean  RndMeth=Simplest  InputSameDT=off
  R_cmp_A2 : RelationalOperator  Operator=>  OutDataTypeStr=boolean  RndMeth=Simplest  InputSameDT=off
  R_cmp_B1 : RelationalOperator  Operator=>  OutDataTypeStr=boolean  RndMeth=Simplest  InputSameDT=off
  R_cmp_B2 : RelationalOperator  Operator=>  OutDataTypeStr=boolean  RndMeth=Simplest  InputSameDT=off
  R_cmp_C1 : RelationalOperator  Operator=>  OutDataTypeStr=boolean  RndMeth=Simplest  InputSameDT=off
  R_cmp_C2 : RelationalOperator  Operator=>  OutDataTypeStr=boolean  RndMeth=Simplest  InputSameDT=off
  R_gate_mux_A : Mux
  R_gate_mux_B : Mux
  R_gate_mux_C : Mux
  R_not_A1 : Logic  Operator=NOT  AllPortsSameDT=off  OutDataTypeStr=boolean
  R_not_A2 : Logic  Operator=NOT  AllPortsSameDT=off  OutDataTypeStr=boolean
  R_not_B1 : Logic  Operator=NOT  AllPortsSameDT=off  OutDataTypeStr=boolean
  R_not_B2 : Logic  Operator=NOT  AllPortsSameDT=off  OutDataTypeStr=boolean
  R_not_C1 : Logic  Operator=NOT  AllPortsSameDT=off  OutDataTypeStr=boolean
  R_not_C2 : Logic  Operator=NOT  AllPortsSameDT=off  OutDataTypeStr=boolean
  m_ref_demux : Demux  Outputs=6
  HBC_A_1 : PMIOPort  Side=Left
  HBC_A_2 : PMIOPort  Port=2  Side=Left
  HBC_B_1 : PMIOPort  Port=3  Side=Left
  HBC_B_2 : PMIOPort  Port=4  Side=Left
  HBC_C_1 : PMIOPort  Port=5  Side=Left
  HBC_C_2 : PMIOPort  Port=6  Side=Left
  DC_pos : PMIOPort  Port=7  Side=Right
  DC_neg : PMIOPort  Port=8  Side=Right
  wires:
  m_ref6/1 -> m_ref_demux/1
  m_ref_demux/1 -> R_cmp_A1/1
  R_carrier_A1/1 -> R_cmp_A1/2
  R_cmp_A1/1 -> R_gate_mux_A/1, R_not_A1/1
  R_not_A1/1 -> R_gate_mux_A/2
  m_ref_demux/2 -> R_cmp_A2/1
  R_carrier_A2/1 -> R_cmp_A2/2
  R_cmp_A2/1 -> R_gate_mux_A/3, R_not_A2/1
  R_not_A2/1 -> R_gate_mux_A/4
  R_gate_mux_A/1 -> R_UB_A/1
  m_ref_demux/3 -> R_cmp_B1/1
  R_carrier_B1/1 -> R_cmp_B1/2
  R_cmp_B1/1 -> R_gate_mux_B/1, R_not_B1/1
  R_not_B1/1 -> R_gate_mux_B/2
  m_ref_demux/4 -> R_cmp_B2/1
  R_carrier_B2/1 -> R_cmp_B2/2
  R_cmp_B2/1 -> R_gate_mux_B/3, R_not_B2/1
  R_not_B2/1 -> R_gate_mux_B/4
  R_gate_mux_B/1 -> R_UB_B/1
  m_ref_demux/5 -> R_cmp_C1/1
  R_carrier_C1/1 -> R_cmp_C1/2
  R_cmp_C1/1 -> R_gate_mux_C/1, R_not_C1/1
  R_not_C1/1 -> R_gate_mux_C/2
  m_ref_demux/6 -> R_cmp_C2/1
  R_carrier_C2/1 -> R_cmp_C2/2
  R_cmp_C2/1 -> R_gate_mux_C/3, R_not_C2/1
  R_not_C2/1 -> R_gate_mux_C/4
  R_gate_mux_C/1 -> R_UB_C/1
  connections:
  HBC_A_1/RConn1 -- R_UB_A/LConn1
  HBC_A_2/RConn1 -- R_UB_A/LConn2
  HBC_B_1/RConn1 -- R_UB_B/LConn1
  HBC_B_2/RConn1 -- R_UB_B/LConn2
  HBC_C_1/RConn1 -- R_UB_C/LConn1
  HBC_C_2/RConn1 -- R_UB_C/LConn2
  R_UB_A/RConn1 -- DC_pos/RConn1 -- R_UB_B/RConn1 -- R_UB_C/RConn1
  R_UB_A/RConn2 -- R_UB_B/RConn2 -- DC_neg/RConn1 -- R_UB_C/RConn2

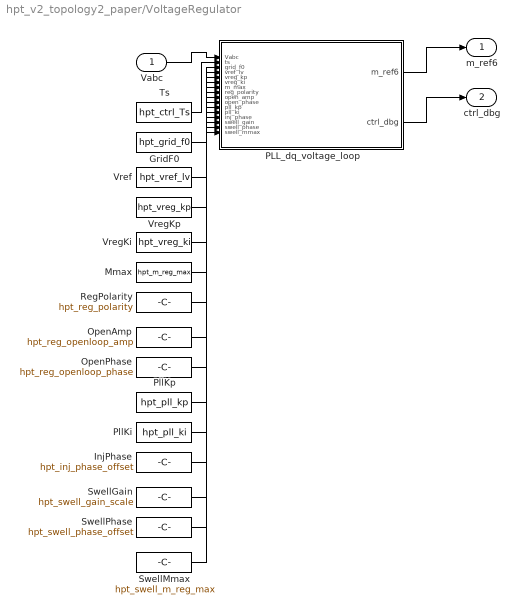
== system hpt_v2_topology2_paper/VoltageRegulator ==
  Vabc : Inport
  GridF0 : Constant  Value=hpt_grid_f0
  InjPhase : Constant  Value=hpt_inj_phase_offset
  Mmax : Constant  Value=hpt_m_reg_max
  OpenAmp : Constant  Value=hpt_reg_openloop_amp
  OpenPhase : Constant  Value=hpt_reg_openloop_phase
  PLL_dq_voltage_loop : MATLAB Function  TreatAsAtomicUnit=on
  PllKi : Constant  Value=hpt_pll_ki
  PllKp : Constant  Value=hpt_pll_kp
  RegPolarity : Constant  Value=hpt_reg_polarity
  SwellGain : Constant  Value=hpt_swell_gain_scale
  SwellMmax : Constant  Value=hpt_swell_m_reg_max
  SwellPhase : Constant  Value=hpt_swell_phase_offset
  Ts : Constant  Value=hpt_ctrl_Ts
  Vref : Constant  Value=hpt_vref_lv
  VregKi : Constant  Value=hpt_vreg_ki
  VregKp : Constant  Value=hpt_vreg_kp
  m_ref6 : Outport
  ctrl_dbg : Outport  Port=2
  wires:
  Ts/1 -> PLL_dq_voltage_loop/2(ts)
  GridF0/1 -> PLL_dq_voltage_loop/3(grid_f0)
  Vref/1 -> PLL_dq_voltage_loop/4(vref_lv)
  VregKp/1 -> PLL_dq_voltage_loop/5(vreg_kp)
  VregKi/1 -> PLL_dq_voltage_loop/6(vreg_ki)
  Mmax/1 -> PLL_dq_voltage_loop/7(m_max)
  RegPolarity/1 -> PLL_dq_voltage_loop/8(reg_polarity)
  OpenAmp/1 -> PLL_dq_voltage_loop/9(open_amp)
  OpenPhase/1 -> PLL_dq_voltage_loop/10(open_phase)
  PllKp/1 -> PLL_dq_voltage_loop/11(pll_kp)
  PllKi/1 -> PLL_dq_voltage_loop/12(pll_ki)
  InjPhase/1 -> PLL_dq_voltage_loop/13(inj_phase)
  SwellGain/1 -> PLL_dq_voltage_loop/14(swell_gain)
  SwellPhase/1 -> PLL_dq_voltage_loop/15(swell_phase)
  SwellMmax/1 -> PLL_dq_voltage_loop/16(swell_mmax)
  Vabc/1 -> PLL_dq_voltage_loop/1(Vabc)
  PLL_dq_voltage_loop/1(m_ref6) -> m_ref6/1
  PLL_dq_voltage_loop/2(ctrl_dbg) -> ctrl_dbg/1

== matlab function hpt_v2_topology2_paper/EnergyController/Vdc_dq_current_loop ==
  data: vdc input; m_abc output; Vabc input; Iabc input; ts input; grid_f0 input; vdc_ref input; vdc_kp input; vdc_ki input; id_max input; cur_kp input; cur_ki input; mmax input; pll_kp input; pll_ki input; vff_gain input; control_sign input; polarity input; dbg output
function [m_abc, dbg] = fcn(vdc, Vabc, Iabc, ts, grid_f0, vdc_ref, vdc_kp, vdc_ki, id_max, cur_kp, cur_ki, mmax, pll_kp, pll_ki, vff_gain, control_sign, polarity)
%#codegen
persistent theta xi_pll xi_vdc xi_id xi_iq t_ctrl vmag_nom hvrt_latch
if isempty(theta)
    theta = 0;
    xi_pll = 0;
    xi_vdc = 0;
    xi_id = 0;
    xi_iq = 0;
    t_ctrl = 0;
    vmag_nom = 0;
    hvrt_latch = 0;
end
t_ctrl = t_ctrl + ts;
va = Vabc(1); vb = Vabc(2); vc = Vabc(3);
ia = Iabc(1); ib = Iabc(2); ic = Iabc(3);
valpha = (2/3) * (va - 0.5*vb - 0.5*vc);
vbeta = (sqrt(3)/3) * (vb - vc);
vmag = sqrt(valpha*valpha + vbeta*vbeta);
if t_ctrl < 0.02
    if vmag_nom == 0; vmag_nom = vmag; else; vmag_nom = 0.98*vmag_nom + 0.02*vmag; end
end
if vmag_nom <= 1; vmag_nom = max(vmag, 1); end
if vdc > 1.35 * vdc_ref
    hvrt_latch = 1;
elseif hvrt_latch >= 0.5 && vmag < 1.01 * vmag_nom && abs(vdc - vdc_ref) < 25
    hvrt_latch = 0;
end
eff_control_sign = control_sign;
eff_polarity = polarity;
if hvrt_latch >= 0.5
    eff_control_sign = abs(control_sign);
    eff_polarity = abs(polarity);
end
ialpha = (2/3) * (ia - 0.5*ib - 0.5*ic);
ibeta = (sqrt(3)/3) * (ib - ic);
theta_meas = atan2(vbeta, valpha);
pll_err = atan2(sin(theta_meas - theta), cos(theta_meas - theta));
xi_pll = xi_pll + pll_ki * pll_err * ts;
omega = 2*pi*grid_f0 + pll_kp * pll_err + xi_pll;
theta = theta + omega * ts;
theta = theta - 2*pi*floor(theta/(2*pi));
ct = cos(theta); st = sin(theta);
vd = valpha*ct + vbeta*st;
vq = -valpha*st + vbeta*ct;
id = ialpha*ct + ibeta*st;
iq = -ialpha*st + ibeta*ct;
err = vdc_ref - vdc;
if abs(err) < 3 || t_ctrl < 0.02
    xi_vdc = 0;
    id_ref = 0;
else
    xi_vdc = xi_vdc + vdc_ki * err * ts;
    id_unsat = vdc_kp * err + xi_vdc;
    id_ref = min(max(id_unsat, -id_max), id_max);
    if id_ref ~= id_unsat
        xi_vdc = id_ref - vdc_kp * err;
    end
end
iq_ref = 0;
eid = id_ref - id;
eiq = iq_ref - iq;
xi_id = xi_id + cur_ki * eid * ts;
xi_iq = xi_iq + cur_ki * eiq * ts;
vd_ctrl = cur_kp * eid + xi_id;
vq_ctrl = cur_kp * eiq + xi_iq;
vconv_d = vff_gain * vd - eff_control_sign * vd_ctrl;
vconv_q = vff_gain * vq - eff_control_sign * vq_ctrl;
conv_alpha = vconv_d*ct - vconv_q*st;
conv_beta = vconv_d*st + vconv_q*ct;
ma_unsat = 2 * conv_alpha / max(abs(vdc), 50);
mb_unsat = 2 * (-0.5*conv_alpha + (sqrt(3)/2)*conv_beta) / max(abs(vdc), 50);
mc_unsat = 2 * (-0.5*conv_alpha - (sqrt(3)/2)*conv_beta) / max(abs(vdc), 50);
ma = min(max(ma_unsat, -mmax), mmax);
mb = min(max(mb_unsat, -mmax), mmax);
mc = min(max(mc_unsat, -mmax), mmax);
if abs(ma) >= mmax || abs(mb) >= mmax || abs(mc) >= mmax
    xi_id = xi_id - cur_ki * eid * ts;
    xi_iq = xi_iq - cur_ki * eiq * ts;
end
m_abc = eff_polarity * [ma; mb; mc];
p_ac = va*ia + vb*ib + vc*ic;
dbg = [theta; vd; vq; id; iq; id_ref; vdc; err; p_ac; ma; mb; mc];
end

== matlab function hpt_v2_topology2_paper/VoltageRegulator/PLL_dq_voltage_loop ==
  data: Vabc input; m_ref6 output; ts input; grid_f0 input; vref_lv input; vreg_kp input; vreg_ki input; m_max input; reg_polarity input; open_amp input; open_phase input; pll_kp input; pll_ki input; inj_phase input; swell_gain input; swell_phase input; swell_mmax input; ctrl_dbg output
function [m_ref6, ctrl_dbg] = fcn(Vabc, ts, grid_f0, vref_lv, vreg_kp, vreg_ki, m_max, reg_polarity, open_amp, open_phase, pll_kp, pll_ki, inj_phase, swell_gain, swell_phase, swell_mmax)
%#codegen
persistent theta xi_pll xi_a xi_b xi_c t_ctrl v_rms_f
if isempty(theta)
    theta = 0;
    xi_pll = 0;
    xi_a = 0;
    xi_b = 0;
    xi_c = 0;
    t_ctrl = 0;
    v_rms_f = 0;
end
t_ctrl = t_ctrl + ts;
m_ref6 = zeros(6, 1);
ctrl_dbg = zeros(7, 1);
va = Vabc(1);
vb = Vabc(2);
vc = Vabc(3);
alpha = (2/3) * (va - 0.5*vb - 0.5*vc);
beta = (sqrt(3)/3) * (vb - vc);
theta_meas = atan2(beta, alpha);
pll_err = atan2(sin(theta_meas - theta), cos(theta_meas - theta));
xi_pll = xi_pll + pll_ki * pll_err * ts;
omega = 2*pi*grid_f0 + pll_kp * pll_err + xi_pll;
theta = theta + omega * ts;
theta = theta - 2*pi*floor(theta/(2*pi));
ct = cos(theta);
st = sin(theta);
vd = alpha*ct + beta*st;
vq = -alpha*st + beta*ct;
v_rms = sqrt(max((va*va + vb*vb + vc*vc) / 3, 0));
if v_rms_f == 0
    v_rms_f = v_rms;
end
alpha_v = min(max(ts / 0.005, 0), 1);
v_rms_f = v_rms_f + alpha_v * (v_rms - v_rms_f);
v_meas = v_rms_f;
if open_amp > 0
    mo = min(max(open_amp, 0), m_max);
    oa = mo*cos(theta + open_phase);
    ob = mo*cos(theta - 2*pi/3 + open_phase);
    oc = mo*cos(theta + 2*pi/3 + open_phase);
    m_amp = sqrt((oa*oa + ob*ob + oc*oc) / 3);
    m_ref6 = reg_polarity * [oa; -oa; ob; -ob; oc; -oc];
    ctrl_dbg = [theta; vd; vq; v_meas; vref_lv - v_meas; m_amp; open_phase];
    return;
end
v_err = vref_lv - v_meas;
err_pu = v_err / max(vref_lv, 1e-6);
phi = inj_phase;
m_limit = m_max;
if abs(err_pu) < 0.002
    kp_eff = 0;
    ki_eff = 0;
    xi_a = 0;
    xi_b = 0;
    xi_c = 0;
    err_eff = 0;
elseif err_pu >= 0
    kp_eff = abs(vreg_kp);
    ki_eff = abs(vreg_ki);
    err_eff = err_pu;
    phi = inj_phase;
    m_limit = m_max;
else
    kp_eff = abs(vreg_kp) * swell_gain;
    ki_eff = abs(vreg_ki) * swell_gain;
    err_eff = err_pu;
    phi = swell_phase;
    m_limit = min(abs(swell_mmax), m_max);
    if kp_eff == 0 && ki_eff == 0
        xi_a = 0;
        xi_b = 0;
        xi_c = 0;
    end
end
if t_ctrl > 0.02
    xi_a = xi_a + ki_eff * err_eff * ts;
else
    xi_a = 0;
end
m_unsat = kp_eff * err_eff + xi_a;
m_cmd = min(max(m_unsat, -m_limit), m_limit);
if m_cmd ~= m_unsat
    xi_a = m_cmd - kp_eff * err_eff;
end
ma = m_cmd * sin(theta + phi);
mb = m_cmd * sin(theta + phi - 2*pi/3);
mc = m_cmd * sin(theta + phi + 2*pi/3);
m_amp = sqrt((ma*ma + mb*mb + mc*mc) / 3);
m_ref6 = reg_polarity * [ma; -ma; mb; -mb; mc; -mc];
ctrl_dbg = [theta; vd; vq; v_meas; v_err; m_amp; phi];
end
